simulink model "cgen_fi"  (R2018a)
settings: Solver=FixedStepDiscrete  StartTime=0.0  StopTime=0  RelTol=1e-3
values from neighbouring files (symbols this model uses):
  b = fidemo.fi_fir_coefficients    [setFIRInputs.m]
  noise = sin(2*pi*2140*(0:n-1)'./Fs)    [setFIRInputs.m]
  x = x + noise    [setFIRInputs.m]
  zi = zeros(length(b),1)    [setFIRInputs.m]
settings Model: Creator=Krishna Bhatia  LastModifiedBy=Krishna Bhatia

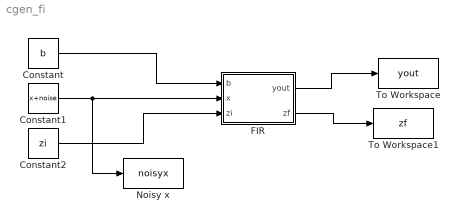
== system cgen_fi ==
  Constant : Constant  Value=b  VectorParams1D=off  OutDataTypeStr=fixdt(1,12,2^-12,0)
  Constant1 : Constant  Value=x+noise  VectorParams1D=off  OutDataTypeStr=fixdt(1,12,2^-8,0)  SampleTime=1
  Constant2 : Constant  Value=zi  VectorParams1D=off  OutDataTypeStr=fixdt(1,12,2^0,0)
  FIR : MATLAB Function  TreatAsAtomicUnit=on
  Noisy x : ToWorkspace  VariableName=noisyx  SampleTime=-1
  To Workspace : ToWorkspace  VariableName=yout  SampleTime=-1
  To Workspace1 : ToWorkspace  VariableName=zf  SampleTime=-1
  wires:
  Constant/1 -> FIR/1(b)
  Constant2/1 -> FIR/3(zi)
  Constant1/1 -> Noisy x/1, FIR/2(x)
  FIR/1(yout) -> To Workspace/1
  FIR/2(zf) -> To Workspace1/1

== matlab function cgen_fi/FIR ==
  settings: fimath=|
      | fimath('RoundingMethod','Floor','OverflowAction','Wrap',...
      |     'ProductMode','KeepLSB','ProductWordLength',32,...
      |     'SumMode','KeepLSB','SumWordLength',32)
  data: b input; yout output; x input; zi input; zf output
function [yout,zf] = dffirdemo(b, x, zi) %#codegen
%codegen_fi doc model example
%Initialize the output signal yout and the final conditions zf
Ty = numerictype(1,12,8);
yout = fi(zeros(size(x)),'numerictype',Ty);
zf = zi;

% FIR filter code
for k=1:length(x);
  % Update the states: z = [x(k);z(1:end-1)]  
  zf(:) = [x(k);zf(1:end-1)];
  % Form the output: y(k) = b*z
  yout(k) = b*zf;
end

% Plot the outputs only in simulation.
% This does not generate C code.
figure;
subplot(211);plot(x); title('Noisy Signal');grid;
subplot(212);plot(yout); title('Filtered Signal');grid;
